simulink model "signalflussalgebra"  (R2015a)
settings: Solver=ode45  StartTime=0.0  StopTime=tsim  RelTol=1e-3
StartFcn:
  | if ~evalin('base','exist(''G2'')')
  |     fprintf('%s unknow!\n','G2')
  | else
  |     G2=evalin('base','G2')
  | end
model workspace (MATLAB code in the model file):
  | if ~evalin('base','exist(''G2'')')
  |     fprintf('%s unknow!\n','G2')
  | else
  |     G2=evalin('base','G2')
  | end
libraries: simulink_extras x2
settings Model: Creator=mainster  LastModifiedBy=mainster
settings SolverCC: AlgebraicLoopSolver=LineSearch

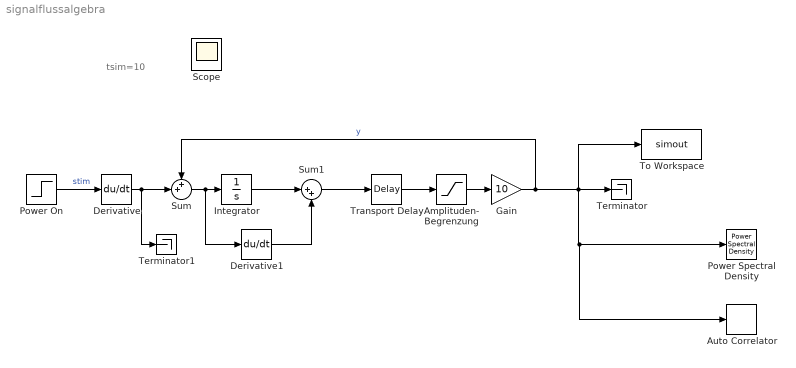
== system signalflussalgebra ==
  note: tsim=10
  Amplituden- Begrenzung : Saturate  UpperLimit=1  LowerLimit=-1
  Auto Correlator : simulink_extras/Additional Sinks/Auto Correlator  npts=100  HowOften=50  sampleT=0.1
  Derivative : Derivative  CoefficientInTFapproximation=100
  Derivative1 : Derivative  CoefficientInTFapproximation=1000
  Gain : Gain  Gain=10
  Integrator : Integrator  InitialCondition=1
  Power On : Step  Time=0.2  SampleTime=0
      settings: AttributesFormatString=|
      | time: %<Time>
      | befor: %<Before>
      | after: %<after>
  Power Spectral Density : simulink_extras/Additional Sinks/Power Spectral Density  npts=128  fftpts=512  HowOften=64  sampleT=0.1
  Sum : Sum  Inputs=++|
  Sum1 : Sum  Inputs=|++
  Terminator : Terminator
  Terminator1 : Terminator
  To Workspace : ToWorkspace  VariableName=simout  SaveFormat=Timeseries  SampleTime=-1
  Transport Delay : TransportDelay  DelayTime=1e-12
      settings: AttributesFormatString=Delay: %<DelayTime>
  Scope : Scope  NumInputPorts=2
      settings: ShowLegends=on  TimeRange=10  YMin=-5~-1.2  YMax=5~1.2
  wires:
  Gain/1 -> Sum/1, To Workspace/1, Auto Correlator/1, Power Spectral Density/1, Terminator/1  "y"
  Sum/1 -> Derivative1/1, Integrator/1
  Sum1/1 -> Transport Delay/1
  Amplituden- Begrenzung/1 -> Gain/1
  Power On/1 -> Derivative/1  "stim"
  Transport Delay/1 -> Amplituden- Begrenzung/1
  Derivative/1 -> Sum/2, Terminator1/1
  Integrator/1 -> Sum1/1
  Derivative1/1 -> Sum1/2
